simulink model "simulation_UCBF_"  (R2022a)
settings: Solver=VariableStepAuto  StartTime=0.0  StopTime=simTime  RelTol=1e-3
values from neighbouring files (symbols this model uses):
  a = 0.1    [setup_UCBF.m]
  ContGainVec = [Kp Kd]    [setup_UCBF.m]
  Icm = 1/2*m*robot_radius^2    (= 0.225)    [setup_UCBF.m]
  m = 5    [setup_UCBF.m]
  mu = 0.3    [setup_UCBF.m]
  obstacles = setup_environment(MAP,a,robot_radius)    [setup_UCBF.m]
  params = [m,Icm,a]    [setup_UCBF.m]
  qg = [6 ; -1]    [setup_UCBF.m]
  qstart = [-2 0 pi/2]'    [setup_UCBF.m]
  vwstart = [0 0]'    [setup_UCBF.m]
undefined symbols (not defined in the file or in its folder): threshold_skip
libraries: slctrlblks x1
settings Model: Creator=mirkomizzoni  LastModifiedBy=dennis

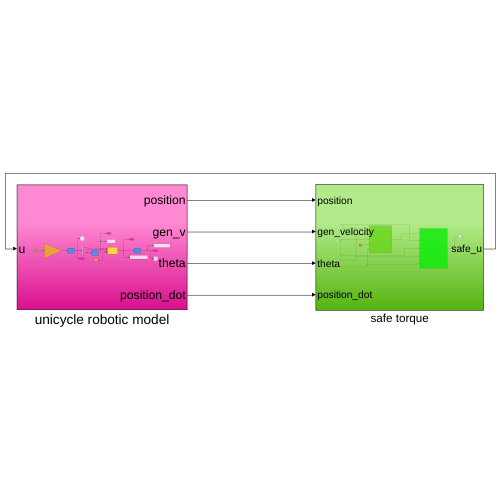
[thumbnail: Simulink's stored preview of the top-level diagram]
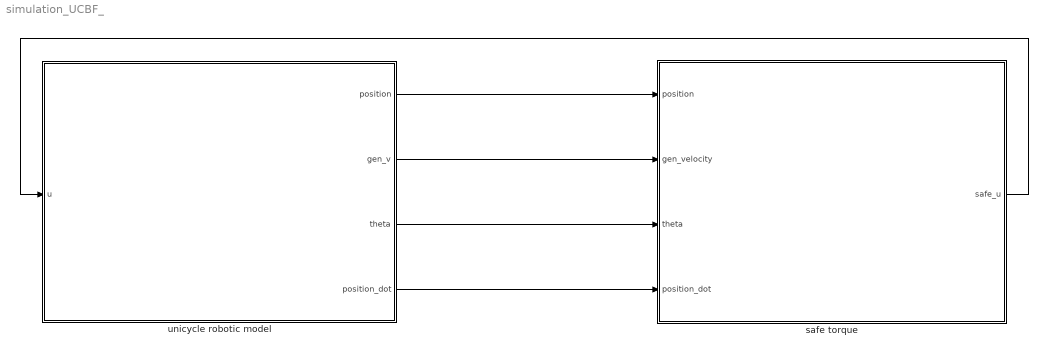
== system simulation_UCBF_ ==
  safe torque : Subsystem
  unicycle robotic model : Subsystem
  wires:
  unicycle robotic model/3(theta) -> safe torque/3(theta)
  unicycle robotic model/2(gen_v) -> safe torque/2(gen_velocity)
  unicycle robotic model/4(position_dot) -> safe torque/4(position_dot)
  unicycle robotic model/1(position) -> safe torque/1(position)
  safe torque/1(safe_u) -> unicycle robotic model/1(u)

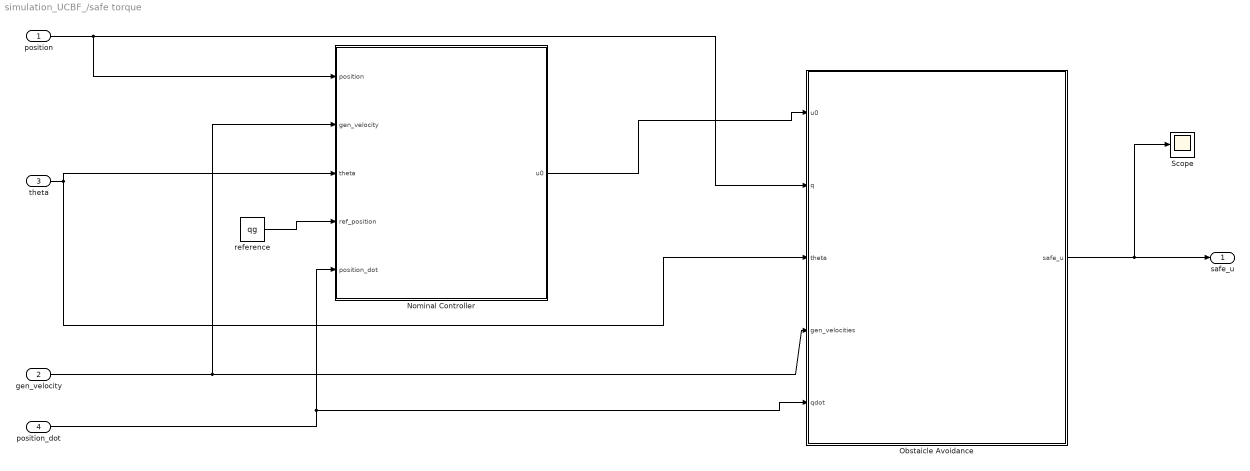
== system simulation_UCBF_/safe torque ==
  position : Inport
  gen_velocity : Inport  Port=2
  theta : Inport  Port=3
  position_dot : Inport  Port=4
  Nominal Controller : Subsystem
  Obstaicle Avoidance : Subsystem
  Scope : Scope
  reference : Constant  Value=qg
  safe_u : Outport
  wires:
  theta/1 -> Nominal Controller/3(theta), Obstaicle Avoidance/3(theta)
  position/1 -> Nominal Controller/1(position), Obstaicle Avoidance/2(q)
  position_dot/1 -> Nominal Controller/5(position_dot), Obstaicle Avoidance/5(qdot)
  gen_velocity/1 -> Nominal Controller/2(gen_velocity), Obstaicle Avoidance/4(gen_velocities)
  reference/1 -> Nominal Controller/4(ref_position)
  Nominal Controller/1(u0) -> Obstaicle Avoidance/1(u0)
  Obstaicle Avoidance/1(safe_u) -> Scope/1, safe_u/1

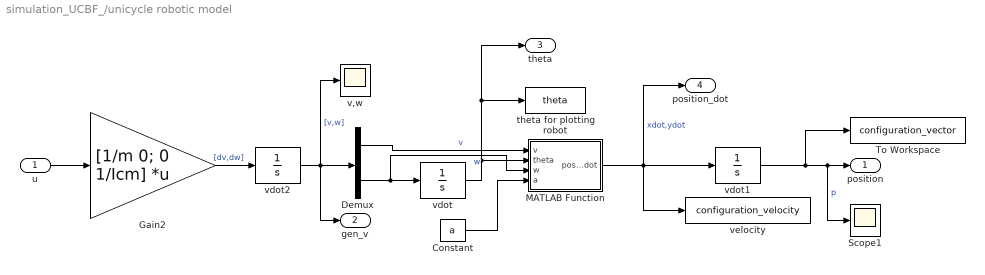
== system simulation_UCBF_/unicycle robotic model ==
  u : Inport
  Constant : Constant  Value=a
  Demux : Demux  Outputs=2
  Gain2 : Gain  Gain=[1/m 0; 0 1/Icm]  Multiplication=Matrix(K*u)
  MATLAB Function : MATLAB Function  TreatAsAtomicUnit=on
  Scope1 : Scope
  To Workspace : ToWorkspace  VariableName=configuration_vector  SaveFormat=Timeseries  SampleTime=0.01
  theta for plotting robot : ToWorkspace  VariableName=theta  SaveFormat=Timeseries  SampleTime=0.01
  v,w : Scope
  vdot : Integrator  InitialCondition=qstart(3)
  vdot1 : Integrator  InitialCondition=qstart(1:2)
  vdot2 : Integrator  InitialCondition=vwstart
  velocity : ToWorkspace  VariableName=configuration_velocity  SaveFormat=Timeseries  SampleTime=0.01
  position : Outport
  gen_v : Outport  Port=2
  theta : Outport  Port=3
  position_dot : Outport  Port=4
  wires:
  u/1 -> Gain2/1
  Gain2/1 -> vdot2/1  "[dv,dw]"
  Demux/2 -> vdot/1, MATLAB Function/3(w)  "w"
  vdot2/1 -> gen_v/1, Demux/1, v,w/1  "[v,w]"
  vdot/1 -> theta/1, theta for plotting robot/1, MATLAB Function/2(theta)
  MATLAB Function/1(positiondot) -> position_dot/1, velocity/1, vdot1/1  "xdot,ydot"
  vdot1/1 -> position/1, Scope1/1, To Workspace/1  "p"
  Demux/1 -> MATLAB Function/1(v)  "v"
  Constant/1 -> MATLAB Function/4(a)

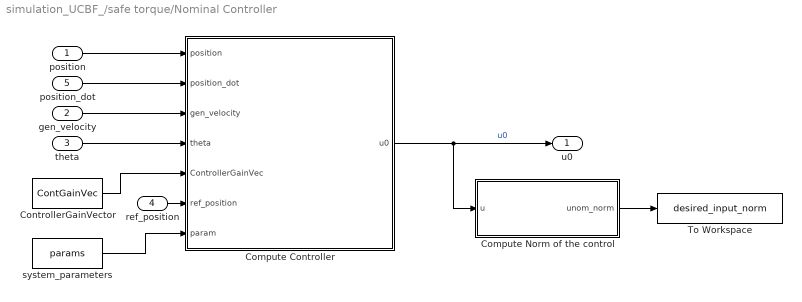
== system simulation_UCBF_/safe torque/Nominal Controller ==
  position : Inport
  gen_velocity : Inport  Port=2
  theta : Inport  Port=3
  ref_position : Inport  Port=4
  position_dot : Inport  Port=5
  Compute Controller : MATLAB Function  TreatAsAtomicUnit=on
  Compute Norm of the control : MATLAB Function  TreatAsAtomicUnit=on
  ControllerGainVector : Constant  Value=ContGainVec
  To Workspace : ToWorkspace  VariableName=desired_input_norm  SaveFormat=Timeseries  SampleTime=0.01
  system_parameters : Constant  Value=params
  u0 : Outport
  wires:
  ref_position/1 -> Compute Controller/6(ref_position)
  ControllerGainVector/1 -> Compute Controller/5(ControllerGainVec)
  Compute Controller/1(u0) -> Compute Norm of the control/1(u), u0/1  "u0"
  position_dot/1 -> Compute Controller/2(position_dot)
  position/1 -> Compute Controller/1(position)
  theta/1 -> Compute Controller/4(theta)
  gen_velocity/1 -> Compute Controller/3(gen_velocity)
  system_parameters/1 -> Compute Controller/7(param)
  Compute Norm of the control/1(unom_norm) -> To Workspace/1

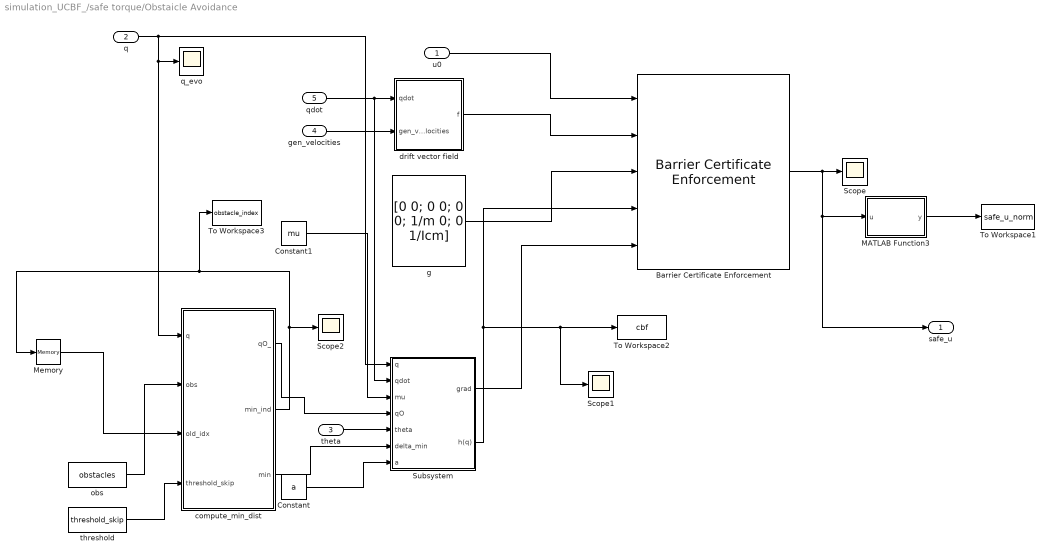
== system simulation_UCBF_/safe torque/Obstaicle Avoidance ==
  u0 : Inport
  q : Inport  Port=2
  theta : Inport  Port=3
  gen_velocities : Inport  Port=4
  qdot : Inport  Port=5
  Barrier Certificate Enforcement : slctrlblks/Barrier Certificate Enforcement  nx=5  nu=2  nc=1  gamma=alpha  beta=1  external_umax=off  external_umin=off  Ts=0.01  maxiter=300  tol=1e-06  output_exitflag=off
      settings: SourceProductBaseCode=SD
  Constant : Constant  Value=a
  Constant1 : Constant  Value=mu
  MATLAB Function3 : MATLAB Function  TreatAsAtomicUnit=on
  Memory : Memory  InitialCondition=1
  Scope : Scope
  Scope1 : Scope
  Scope2 : Scope
  Subsystem : Subsystem
  To Workspace1 : ToWorkspace  VariableName=safe_u_norm  SaveFormat=Timeseries  SampleTime=0.01
  To Workspace2 : ToWorkspace  VariableName=cbf  SaveFormat=Timeseries  SampleTime=0.01
  To Workspace3 : ToWorkspace  VariableName=obstacle_index  SaveFormat=Timeseries  SampleTime=0.01
  compute_min_dist : MATLAB Function  TreatAsAtomicUnit=on
  drift vector field : MATLAB Function  TreatAsAtomicUnit=on
  g : Constant  Value=[0 0; 0 0; 0 0; 1/m 0; 0 1/Icm]  VectorParams1D=off
  obs : Constant  Value=obstacles  VectorParams1D=off
  q_evo : Scope
  threshold : Constant  Value=threshold_skip  VectorParams1D=off
  safe_u : Outport
  wires:
  q/1 -> Subsystem/1(q), q_evo/1, compute_min_dist/1(q)
  qdot/1 -> Subsystem/2(qdot), drift vector field/1(qdot)
  MATLAB Function3/1(y) -> To Workspace1/1
  threshold/1 -> compute_min_dist/4(threshold_skip)
  u0/1 -> Barrier Certificate Enforcement/1
  obs/1 -> compute_min_dist/2(obs)
  Memory/1 -> compute_min_dist/3(old_idx)
  drift vector field/1(f) -> Barrier Certificate Enforcement/2
  Barrier Certificate Enforcement/1 -> Scope/1, safe_u/1, MATLAB Function3/1(u)
  compute_min_dist/2(min_ind) -> Scope2/1, To Workspace3/1, Memory/1
  g/1 -> Barrier Certificate Enforcement/3
  gen_velocities/1 -> drift vector field/2(gen_velocities)
  Subsystem/2(h(q)) -> Barrier Certificate Enforcement/4, Scope1/1, To Workspace2/1
  Constant1/1 -> Subsystem/3(mu)
  compute_min_dist/1(qO_) -> Subsystem/4(qO)
  theta/1 -> Subsystem/5(theta)
  compute_min_dist/3(min) -> Subsystem/6(delta_min)
  Constant/1 -> Subsystem/7(a)
  Subsystem/1(grad) -> Barrier Certificate Enforcement/5

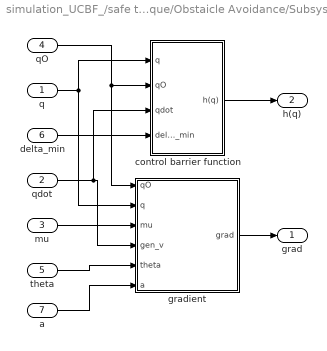
== system simulation_UCBF_/safe torque/Obstaicle Avoidance/Subsystem ==
  q : Inport
  qdot : Inport  Port=2
  mu : Inport  Port=3
  qO : Inport  Port=4
  theta : Inport  Port=5
  delta_min : Inport  Port=6
  a : Inport  Port=7
  control barrier function : Subsystem
  gradient : MATLAB Function  TreatAsAtomicUnit=on
  grad : Outport
  h(q) : Outport  Port=2
  wires:
  qdot/1 -> control barrier function/3(qdot), gradient/4(gen_v)
  q/1 -> control barrier function/1(q), gradient/2(q)
  qO/1 -> gradient/1(qO), control barrier function/2(qO)
  delta_min/1 -> control barrier function/4(delta_min)
  control barrier function/1(h(q)) -> h(q)/1
  theta/1 -> gradient/5(theta)
  mu/1 -> gradient/3(mu)
  a/1 -> gradient/6(a)
  gradient/1(grad) -> grad/1

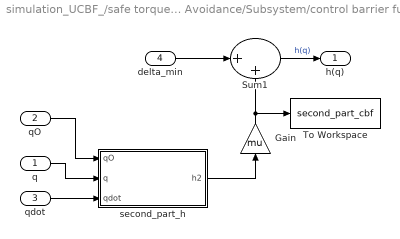
== system simulation_UCBF_/safe torque/Obstaicle Avoidance/Subsystem/control barrier function ==
  q : Inport
  qO : Inport  Port=2
  qdot : Inport  Port=3
  delta_min : Inport  Port=4
  Gain : Gain  Gain=mu
  Sum1 : Sum  Inputs=|++
  To Workspace : ToWorkspace  VariableName=second_part_cbf  SaveFormat=Timeseries  SampleTime=0.01
  second_part_h : MATLAB Function  TreatAsAtomicUnit=on
  h(q) : Outport
  wires:
  q/1 -> second_part_h/2(q)
  second_part_h/1(h2) -> Gain/1
  qdot/1 -> second_part_h/3(qdot)
  Sum1/1 -> h(q)/1  "h(q)"
  delta_min/1 -> Sum1/1
  Gain/1 -> To Workspace/1, Sum1/2
  qO/1 -> second_part_h/1(qO)

== matlab function simulation_UCBF_/safe torque/Nominal Controller/Compute Controller ==
  data: u0 output; position input; position_dot input; gen_velocity input; theta input; ControllerGainVec input; ref_position input; param input
function u0 = posdot(position,position_dot,gen_velocity,theta,ControllerGainVec,ref_position,param)
       v = gen_velocity(1);
       w = gen_velocity(2);
       m = param(1);
       Icm = param(2);
       a = param(3);
       g = [cos(theta)/m, -a*sin(theta)/Icm ; sin(theta)/m, a*cos(theta)/Icm];
       f = [-v*w*sin(theta)-w^2*a*cos(theta); v*w*cos(theta)-w^2*a*sin(theta)];
       kp = ControllerGainVec(1)*eye(2);
       kd = ControllerGainVec(2)*eye(2);
       % vbar is the PD controller
       vbar = kp*(ref_position-position)-kd*position_dot;
       u0 = g\(-f+vbar);
end

== matlab function simulation_UCBF_/safe torque/Nominal Controller/Compute Norm of the control ==
  data: unom_norm output; u input
function unom_norm = norm_control(u)
    unom_norm = norm(u);
end

== matlab function simulation_UCBF_/safe torque/Obstaicle Avoidance/compute_min_dist ==
  data: q input; obs input; qO_ output; min_ind output; old_idx input; threshold_skip input; min output
function [qO_,min_ind,min] = min_dist(q, obs, old_idx, threshold_skip)
    [~,n] = size(obs);
    o1 = obs(:,1);
    min_ind = 1;
    min = norm_obs(q,o1);
    for i=2:n
        oi = obs(:,i);
        t = norm_obs(q,oi);
        if t<min
            min_ind = i;
            min = t;
        end
    end
    oold = obs(:,old_idx);
    old_dist = norm_obs(q,oold);
    if abs(old_dist-min) < threshold_skip
        min_ind = old_idx;
        min = old_dist;
    end
    qO = obs(:,min_ind);
    qO_ = qO(1:2);
end

function min = norm_obs(q, obs)
    min = norm(q-obs(1:2))-obs(3)-obs(4);
end

== matlab function simulation_UCBF_/safe torque/Obstaicle Avoidance/MATLAB Function3 ==
  data: u input; y output
function y = norm_func(u)
    y = norm(u);
end

== matlab function simulation_UCBF_/safe torque/Obstaicle Avoidance/Subsystem/control barrier function/second_part_h ==
  data: qO input; h2 output; q input; qdot input
function h2 = second_part_h(qO,q,qdot)
   h2 = (q-qO)'*qdot;
end

== matlab function simulation_UCBF_/safe torque/Obstaicle Avoidance/drift vector field ==
  data: qdot input; f output; gen_velocities input
function f = make_f(qdot, gen_velocities)
    w = gen_velocities(2);
    f = [qdot; w; 0; 0];
end

== matlab function simulation_UCBF_/safe torque/Obstaicle Avoidance/Subsystem/gradient ==
  data: qO input; grad output; q input; mu input; gen_v input; theta input; a input
function grad = gradient(qO,q, mu, gen_v, theta, a)
    % x y ox oy theta mu a w v 
    ox = qO(1);
    oy = qO(2);
    x = q(1);
    y = q(2);
    v = gen_v(1);
    w = gen_v(2);
%     grad = [2*x - 2*ox + mu*(v*cos(theta) - a*w*sin(theta)), ... 
%         2*y - 2*oy + mu*(v*sin(theta) + a*w*cos(theta)),  ...
%         mu*(v*sin(theta) + a*w*cos(theta))*(ox - x) - mu*(v*cos(theta) - a*w*sin(theta))*(oy - y), ...
%         - mu*cos(theta)*(ox - x) - mu*sin(theta)*(oy - y), ...
%         a*mu*sin(theta)*(ox - x) - a*mu*cos(theta)*(oy - y)]; 

grad=[2*x - 2*ox + mu*(v*cos(theta) - a*w*sin(theta)),...
    2*y - 2*oy + mu*(v*sin(theta) + a*w*cos(theta)), ...
    mu*(v*sin(theta) + a*w*cos(theta))*(ox - x) - mu*(v*cos(theta) - a*w*sin(theta))*(oy - y),...
    - mu*cos(theta)*(ox - x) - mu*sin(theta)*(oy - y),...
    a*mu*sin(theta)*(ox - x) - a*mu*cos(theta)*(oy - y)];

end

== matlab function simulation_UCBF_/unicycle robotic model/MATLAB Function ==
  data: v input; positiondot output; theta input; w input; a input
function positiondot = posdot(v,theta,w,a)
        dx = v*cos(theta)-w*a*sin(theta);
        dy = v*sin(theta)+w*a*cos(theta);
        positiondot = [dx; dy];
end
